simulink model "RBDmodel_unprotected"  (R2023a)
settings: Solver=ode15s  StartTime=0.0  StopTime=10  FixedStep=0.0001  RelTol=1e-3  AbsTol=1e-3  EnableMultiTasking=on
model workspace (MAT data in the model file):
  C_Gimbal = 0.1
  C_IAP = 0.01
  IAP_Pa = 0
  K_Gimbal = 0
  K_IAP = 0
  Left_EO = 0
  Left_IO = 0
  Left_MF = 0
  Left_RA = 0
  Moment_AR = 0
  Moment_FE = 7.5
  Moment_LB = 0
  Right_EO = 0
  Right_IO = 0
  Right_MF = 0
  Right_RA = 0
  a = 1
  b = 1
  muscle_color = [0 0 1]
  muscle_radius = 1
undefined symbols (not defined in the file): X, Y, Z
libraries: nesl_utility x346, sm_lib x329, simulink_extras x33, checkpacklib x3, simulink x1
(part 12 of 13)

== system RBDmodel_unprotected/subsystem/Segmental Moment-Rotation setup/L5-S1 AR setup ==
  Gain3 : Gain  Gain=-1
  Gain8 : Gain
  PS-Simulink Converter : nesl_utility/PS-Simulink Converter  PhysicalDomain=network_engine_domain  SubClassName=ps_output  LeftPortType=input  RightPortType=output  PseudoPeriodic=off  Frequencies=[]  VectorFormat=1-D array  Unit=rad  AffineConversion=off
  PS-Simulink Converter7 : nesl_utility/PS-Simulink Converter  PhysicalDomain=network_engine_domain  SubClassName=ps_output  LeftPortType=input  RightPortType=output  PseudoPeriodic=off  Frequencies=[]  VectorFormat=1-D array  Unit=N*m  AffineConversion=off
  Radians to Degrees : simulink_extras/Transformations/Radians to Degrees
  Moment : PMIOPort  Side=Left
  Rotation : PMIOPort  Port=2  Side=Left
  L5-S1 AR Simscape Rotation : Outport
  L5-S1 AR Simscape Moment : Outport  Port=2
  wires:
  Gain8/1 -> L5-S1 AR Simscape Moment/1  "L5-S1 AR Simscape Moment"
  PS-Simulink Converter7/1 -> Gain8/1
  Radians to Degrees/1 -> Gain3/1
  PS-Simulink Converter/1 -> Radians to Degrees/1
  Gain3/1 -> L5-S1 AR Simscape Rotation/1  "L5-S1 AR Simscape Rotation"
  connections:
  Rotation/RConn1 -- PS-Simulink Converter/LConn1
  Moment/RConn1 -- PS-Simulink Converter7/LConn1

== system RBDmodel_unprotected/subsystem/Segmental Moment-Rotation setup/L5-S1 FE setup ==
  Gain3 : Gain  Gain=-1
  Gain8 : Gain
  PS-Simulink Converter : nesl_utility/PS-Simulink Converter  PhysicalDomain=network_engine_domain  SubClassName=ps_output  LeftPortType=input  RightPortType=output  PseudoPeriodic=off  Frequencies=[]  VectorFormat=1-D array  Unit=rad  AffineConversion=off
  PS-Simulink Converter7 : nesl_utility/PS-Simulink Converter  PhysicalDomain=network_engine_domain  SubClassName=ps_output  LeftPortType=input  RightPortType=output  PseudoPeriodic=off  Frequencies=[]  VectorFormat=1-D array  Unit=N*m  AffineConversion=off
  Radians to Degrees : simulink_extras/Transformations/Radians to Degrees
  Moment : PMIOPort  Side=Left
  Rotation : PMIOPort  Port=2  Side=Left
  L5-S1 FE Simscape Rotation : Outport
  L5-S1 FE Simscape Moment : Outport  Port=2
  wires:
  Radians to Degrees/1 -> Gain3/1
  PS-Simulink Converter/1 -> Radians to Degrees/1
  PS-Simulink Converter7/1 -> Gain8/1
  Gain8/1 -> L5-S1 FE Simscape Moment/1  "L5-S1 FE Simscape Moment"
  Gain3/1 -> L5-S1 FE Simscape Rotation/1  "L5-S1 FE Simscape Rotation"
  connections:
  Rotation/RConn1 -- PS-Simulink Converter/LConn1
  Moment/RConn1 -- PS-Simulink Converter7/LConn1

== system RBDmodel_unprotected/subsystem/Segmental Moment-Rotation setup/L5-S1 LB setup ==
  Gain3 : Gain
  Gain8 : Gain  Gain=-1
  PS-Simulink Converter : nesl_utility/PS-Simulink Converter  PhysicalDomain=network_engine_domain  SubClassName=ps_output  LeftPortType=input  RightPortType=output  PseudoPeriodic=off  Frequencies=[]  VectorFormat=1-D array  Unit=rad  AffineConversion=off
  PS-Simulink Converter7 : nesl_utility/PS-Simulink Converter  PhysicalDomain=network_engine_domain  SubClassName=ps_output  LeftPortType=input  RightPortType=output  PseudoPeriodic=off  Frequencies=[]  VectorFormat=1-D array  Unit=N*m  AffineConversion=off
  Radians to Degrees : simulink_extras/Transformations/Radians to Degrees
  Moment : PMIOPort  Side=Left
  Rotation : PMIOPort  Port=2  Side=Left
  L5-S1 LB Simscape Rotation : Outport
  L5-S1 LB Simscape Moment : Outport  Port=2
  wires:
  Gain8/1 -> L5-S1 LB Simscape Moment/1  "L5-S1 LB Simscape Moment"
  PS-Simulink Converter/1 -> Radians to Degrees/1
  Radians to Degrees/1 -> Gain3/1
  Gain3/1 -> L5-S1 LB Simscape Rotation/1  "L5-S1 LB Simscape Rotation"
  PS-Simulink Converter7/1 -> Gain8/1
  connections:
  Moment/RConn1 -- PS-Simulink Converter7/LConn1
  Rotation/RConn1 -- PS-Simulink Converter/LConn1

== system RBDmodel_unprotected/subsystem/Segmental Moment-Rotation setup/Subsystem ==
  Gain3 : Gain  Gain=-1
  Gain8 : Gain
  PS-Simulink Converter : nesl_utility/PS-Simulink Converter  PhysicalDomain=network_engine_domain  SubClassName=ps_output  LeftPortType=input  RightPortType=output  PseudoPeriodic=off  Frequencies=[]  VectorFormat=1-D array  Unit=rad  AffineConversion=off
  PS-Simulink Converter7 : nesl_utility/PS-Simulink Converter  PhysicalDomain=network_engine_domain  SubClassName=ps_output  LeftPortType=input  RightPortType=output  PseudoPeriodic=off  Frequencies=[]  VectorFormat=1-D array  Unit=N*m  AffineConversion=off
  Radians to Degrees : simulink_extras/Transformations/Radians to Degrees
  Moment : PMIOPort  Side=Left
  Rotation : PMIOPort  Port=2  Side=Left
  L4-L5 FE Simscape Rotation : Outport
  L4-L5 FE Simscape Moment : Outport  Port=2
  wires:
  Radians to Degrees/1 -> Gain3/1
  PS-Simulink Converter/1 -> Radians to Degrees/1
  Gain8/1 -> L4-L5 FE Simscape Moment/1  "L4-L5 FE Simscape Moment"
  PS-Simulink Converter7/1 -> Gain8/1
  Gain3/1 -> L4-L5 FE Simscape Rotation/1  "L4-L5 FE Simscape Rotation"
  connections:
  Moment/RConn1 -- PS-Simulink Converter7/LConn1
  Rotation/RConn1 -- PS-Simulink Converter/LConn1

== system RBDmodel_unprotected/subsystem/Segmental Moment-Rotation setup/Subsystem1 ==
  Gain3 : Gain
  Gain8 : Gain  Gain=-1
  PS-Simulink Converter : nesl_utility/PS-Simulink Converter  PhysicalDomain=network_engine_domain  SubClassName=ps_output  LeftPortType=input  RightPortType=output  PseudoPeriodic=off  Frequencies=[]  VectorFormat=1-D array  Unit=rad  AffineConversion=off
  PS-Simulink Converter7 : nesl_utility/PS-Simulink Converter  PhysicalDomain=network_engine_domain  SubClassName=ps_output  LeftPortType=input  RightPortType=output  PseudoPeriodic=off  Frequencies=[]  VectorFormat=1-D array  Unit=N*m  AffineConversion=off
  Radians to Degrees : simulink_extras/Transformations/Radians to Degrees
  Moment : PMIOPort  Side=Left
  Rotation : PMIOPort  Port=2  Side=Left
  L4-L5 LB Simscape Rotation : Outport
  L4-L5 LB Simscape Moment : Outport  Port=2
  wires:
  PS-Simulink Converter/1 -> Radians to Degrees/1
  Gain3/1 -> L4-L5 LB Simscape Rotation/1  "L4-L5 LB Simscape Rotation"
  Radians to Degrees/1 -> Gain3/1
  PS-Simulink Converter7/1 -> Gain8/1
  Gain8/1 -> L4-L5 LB Simscape Moment/1  "L4-L5 LB Simscape Moment"
  connections:
  Rotation/RConn1 -- PS-Simulink Converter/LConn1
  Moment/RConn1 -- PS-Simulink Converter7/LConn1

== system RBDmodel_unprotected/subsystem/Segmental Moment-Rotation setup/Subsystem10 ==
  Gain3 : Gain
  Gain8 : Gain  Gain=-1
  PS-Simulink Converter : nesl_utility/PS-Simulink Converter  PhysicalDomain=network_engine_domain  SubClassName=ps_output  LeftPortType=input  RightPortType=output  PseudoPeriodic=off  Frequencies=[]  VectorFormat=1-D array  Unit=rad  AffineConversion=off
  PS-Simulink Converter7 : nesl_utility/PS-Simulink Converter  PhysicalDomain=network_engine_domain  SubClassName=ps_output  LeftPortType=input  RightPortType=output  PseudoPeriodic=off  Frequencies=[]  VectorFormat=1-D array  Unit=N*m  AffineConversion=off
  Radians to Degrees : simulink_extras/Transformations/Radians to Degrees
  Moment : PMIOPort  Side=Left
  Rotation : PMIOPort  Port=2  Side=Left
  L1-L2 LB Simscape Rotation : Outport
  L1-L2 LB Simscape Moment : Outport  Port=2
  wires:
  Radians to Degrees/1 -> Gain3/1
  PS-Simulink Converter/1 -> Radians to Degrees/1
  PS-Simulink Converter7/1 -> Gain8/1
  Gain3/1 -> L1-L2 LB Simscape Rotation/1  "L1-L2 LB Simscape Rotation"
  Gain8/1 -> L1-L2 LB Simscape Moment/1  "L1-L2 LB Simscape Moment"
  connections:
  Moment/RConn1 -- PS-Simulink Converter7/LConn1
  Rotation/RConn1 -- PS-Simulink Converter/LConn1

== system RBDmodel_unprotected/subsystem/Segmental Moment-Rotation setup/Subsystem11 ==
  Gain3 : Gain  Gain=-1
  Gain8 : Gain
  PS-Simulink Converter : nesl_utility/PS-Simulink Converter  PhysicalDomain=network_engine_domain  SubClassName=ps_output  LeftPortType=input  RightPortType=output  PseudoPeriodic=off  Frequencies=[]  VectorFormat=1-D array  Unit=rad  AffineConversion=off
  PS-Simulink Converter7 : nesl_utility/PS-Simulink Converter  PhysicalDomain=network_engine_domain  SubClassName=ps_output  LeftPortType=input  RightPortType=output  PseudoPeriodic=off  Frequencies=[]  VectorFormat=1-D array  Unit=N*m  AffineConversion=off
  Radians to Degrees : simulink_extras/Transformations/Radians to Degrees
  Moment : PMIOPort  Side=Left
  Rotation : PMIOPort  Port=2  Side=Left
  L1-L2 AR Simscape Rotation : Outport
  L1-L2 AR Simscape Moment : Outport  Port=2
  wires:
  Gain3/1 -> L1-L2 AR Simscape Rotation/1  "L1-L2 AR Simscape Rotation"
  Radians to Degrees/1 -> Gain3/1
  PS-Simulink Converter/1 -> Radians to Degrees/1
  PS-Simulink Converter7/1 -> Gain8/1
  Gain8/1 -> L1-L2 AR Simscape Moment/1  "L1-L2 AR Simscape Moment"
  connections:
  Moment/RConn1 -- PS-Simulink Converter7/LConn1
  Rotation/RConn1 -- PS-Simulink Converter/LConn1

== system RBDmodel_unprotected/subsystem/Segmental Moment-Rotation setup/Subsystem2 ==
  Gain3 : Gain  Gain=-1
  Gain8 : Gain
  PS-Simulink Converter : nesl_utility/PS-Simulink Converter  PhysicalDomain=network_engine_domain  SubClassName=ps_output  LeftPortType=input  RightPortType=output  PseudoPeriodic=off  Frequencies=[]  VectorFormat=1-D array  Unit=rad  AffineConversion=off
  PS-Simulink Converter7 : nesl_utility/PS-Simulink Converter  PhysicalDomain=network_engine_domain  SubClassName=ps_output  LeftPortType=input  RightPortType=output  PseudoPeriodic=off  Frequencies=[]  VectorFormat=1-D array  Unit=N*m  AffineConversion=off
  Radians to Degrees : simulink_extras/Transformations/Radians to Degrees
  Moment : PMIOPort  Side=Left
  Rotation : PMIOPort  Port=2  Side=Left
  L4-L5 AR Simscape Rotation : Outport
  L4-L5 AR Simscape Moment : Outport  Port=2
  wires:
  PS-Simulink Converter7/1 -> Gain8/1
  Radians to Degrees/1 -> Gain3/1
  Gain8/1 -> L4-L5 AR Simscape Moment/1  "L4-L5 AR Simscape Moment"
  PS-Simulink Converter/1 -> Radians to Degrees/1
  Gain3/1 -> L4-L5 AR Simscape Rotation/1  "L4-L5 AR Simscape Rotation"
  connections:
  Moment/RConn1 -- PS-Simulink Converter7/LConn1
  Rotation/RConn1 -- PS-Simulink Converter/LConn1

== system RBDmodel_unprotected/subsystem/Segmental Moment-Rotation setup/Subsystem3 ==
  Gain3 : Gain  Gain=-1
  Gain8 : Gain
  PS-Simulink Converter : nesl_utility/PS-Simulink Converter  PhysicalDomain=network_engine_domain  SubClassName=ps_output  LeftPortType=input  RightPortType=output  PseudoPeriodic=off  Frequencies=[]  VectorFormat=1-D array  Unit=rad  AffineConversion=off
  PS-Simulink Converter7 : nesl_utility/PS-Simulink Converter  PhysicalDomain=network_engine_domain  SubClassName=ps_output  LeftPortType=input  RightPortType=output  PseudoPeriodic=off  Frequencies=[]  VectorFormat=1-D array  Unit=N*m  AffineConversion=off
  Radians to Degrees : simulink_extras/Transformations/Radians to Degrees
  Moment : PMIOPort  Side=Left
  Rotation : PMIOPort  Port=2  Side=Left
  L3-L4 FE Simscape Rotation : Outport
  L3-L4 FE Simscape Moment : Outport  Port=2
  wires:
  Radians to Degrees/1 -> Gain3/1
  Gain3/1 -> L3-L4 FE Simscape Rotation/1  "L3-L4 FE Simscape Rotation"
  PS-Simulink Converter/1 -> Radians to Degrees/1
  PS-Simulink Converter7/1 -> Gain8/1
  Gain8/1 -> L3-L4 FE Simscape Moment/1  "L3-L4 FE Simscape Moment"
  connections:
  Moment/RConn1 -- PS-Simulink Converter7/LConn1
  Rotation/RConn1 -- PS-Simulink Converter/LConn1

== system RBDmodel_unprotected/subsystem/Segmental Moment-Rotation setup/Subsystem4 ==
  Gain3 : Gain
  Gain8 : Gain  Gain=-1
  PS-Simulink Converter : nesl_utility/PS-Simulink Converter  PhysicalDomain=network_engine_domain  SubClassName=ps_output  LeftPortType=input  RightPortType=output  PseudoPeriodic=off  Frequencies=[]  VectorFormat=1-D array  Unit=rad  AffineConversion=off
  PS-Simulink Converter7 : nesl_utility/PS-Simulink Converter  PhysicalDomain=network_engine_domain  SubClassName=ps_output  LeftPortType=input  RightPortType=output  PseudoPeriodic=off  Frequencies=[]  VectorFormat=1-D array  Unit=N*m  AffineConversion=off
  Radians to Degrees : simulink_extras/Transformations/Radians to Degrees
  Moment : PMIOPort  Side=Left
  Rotation : PMIOPort  Port=2  Side=Left
  L3-L4 LB Simscape Rotation : Outport
  L3-L4 LB Simscape Moment : Outport  Port=2
  wires:
  Gain8/1 -> L3-L4 LB Simscape Moment/1  "L3-L4 LB Simscape Moment"
  Radians to Degrees/1 -> Gain3/1
  PS-Simulink Converter/1 -> Radians to Degrees/1
  PS-Simulink Converter7/1 -> Gain8/1
  Gain3/1 -> L3-L4 LB Simscape Rotation/1  "L3-L4 LB Simscape Rotation"
  connections:
  Moment/RConn1 -- PS-Simulink Converter7/LConn1
  Rotation/RConn1 -- PS-Simulink Converter/LConn1

== system RBDmodel_unprotected/subsystem/Segmental Moment-Rotation setup/Subsystem5 ==
  Gain3 : Gain  Gain=-1
  Gain8 : Gain
  PS-Simulink Converter : nesl_utility/PS-Simulink Converter  PhysicalDomain=network_engine_domain  SubClassName=ps_output  LeftPortType=input  RightPortType=output  PseudoPeriodic=off  Frequencies=[]  VectorFormat=1-D array  Unit=rad  AffineConversion=off
  PS-Simulink Converter7 : nesl_utility/PS-Simulink Converter  PhysicalDomain=network_engine_domain  SubClassName=ps_output  LeftPortType=input  RightPortType=output  PseudoPeriodic=off  Frequencies=[]  VectorFormat=1-D array  Unit=N*m  AffineConversion=off
  Radians to Degrees : simulink_extras/Transformations/Radians to Degrees
  Moment : PMIOPort  Side=Left
  Rotation : PMIOPort  Port=2  Side=Left
  L3-L4 AR Simscape Rotation : Outport
  L3-L4 AR Simscape Moment : Outport  Port=2
  wires:
  PS-Simulink Converter/1 -> Radians to Degrees/1
  Gain8/1 -> L3-L4 AR Simscape Moment/1  "L3-L4 AR Simscape Moment"
  PS-Simulink Converter7/1 -> Gain8/1
  Radians to Degrees/1 -> Gain3/1
  Gain3/1 -> L3-L4 AR Simscape Rotation/1  "L3-L4 AR Simscape Rotation"
  connections:
  Moment/RConn1 -- PS-Simulink Converter7/LConn1
  Rotation/RConn1 -- PS-Simulink Converter/LConn1

== system RBDmodel_unprotected/subsystem/Segmental Moment-Rotation setup/Subsystem6 ==
  Gain3 : Gain  Gain=-1
  Gain8 : Gain
  PS-Simulink Converter : nesl_utility/PS-Simulink Converter  PhysicalDomain=network_engine_domain  SubClassName=ps_output  LeftPortType=input  RightPortType=output  PseudoPeriodic=off  Frequencies=[]  VectorFormat=1-D array  Unit=rad  AffineConversion=off
  PS-Simulink Converter7 : nesl_utility/PS-Simulink Converter  PhysicalDomain=network_engine_domain  SubClassName=ps_output  LeftPortType=input  RightPortType=output  PseudoPeriodic=off  Frequencies=[]  VectorFormat=1-D array  Unit=N*m  AffineConversion=off
  Radians to Degrees : simulink_extras/Transformations/Radians to Degrees
  Moment : PMIOPort  Side=Left
  Rotation : PMIOPort  Port=2  Side=Left
  L2-L3 FE Simscape Rotation : Outport
  L2-L3 FE Simscape Moment : Outport  Port=2
  wires:
  Gain3/1 -> L2-L3 FE Simscape Rotation/1  "L2-L3 FE Simscape Rotation"
  PS-Simulink Converter/1 -> Radians to Degrees/1
  PS-Simulink Converter7/1 -> Gain8/1
  Radians to Degrees/1 -> Gain3/1
  Gain8/1 -> L2-L3 FE Simscape Moment/1  "L2-L3 FE Simscape Moment"
  connections:
  Rotation/RConn1 -- PS-Simulink Converter/LConn1
  Moment/RConn1 -- PS-Simulink Converter7/LConn1

== system RBDmodel_unprotected/subsystem/Segmental Moment-Rotation setup/Subsystem7 ==
  Gain3 : Gain
  Gain8 : Gain  Gain=-1
  PS-Simulink Converter : nesl_utility/PS-Simulink Converter  PhysicalDomain=network_engine_domain  SubClassName=ps_output  LeftPortType=input  RightPortType=output  PseudoPeriodic=off  Frequencies=[]  VectorFormat=1-D array  Unit=rad  AffineConversion=off
  PS-Simulink Converter7 : nesl_utility/PS-Simulink Converter  PhysicalDomain=network_engine_domain  SubClassName=ps_output  LeftPortType=input  RightPortType=output  PseudoPeriodic=off  Frequencies=[]  VectorFormat=1-D array  Unit=N*m  AffineConversion=off
  Radians to Degrees : simulink_extras/Transformations/Radians to Degrees
  Moment : PMIOPort  Side=Left
  Rotation : PMIOPort  Port=2  Side=Left
  L2-L3 LB Simscape Rotation : Outport
  L2-L3 LB Simscape Moment : Outport  Port=2
  wires:
  PS-Simulink Converter7/1 -> Gain8/1
  PS-Simulink Converter/1 -> Radians to Degrees/1
  Radians to Degrees/1 -> Gain3/1
  Gain3/1 -> L2-L3 LB Simscape Rotation/1  "L2-L3 LB Simscape Rotation"
  Gain8/1 -> L2-L3 LB Simscape Moment/1  "L2-L3 LB Simscape Moment"
  connections:
  Rotation/RConn1 -- PS-Simulink Converter/LConn1
  Moment/RConn1 -- PS-Simulink Converter7/LConn1

== system RBDmodel_unprotected/subsystem/Segmental Moment-Rotation setup/Subsystem8 ==
  Gain3 : Gain  Gain=-1
  Gain8 : Gain
  PS-Simulink Converter : nesl_utility/PS-Simulink Converter  PhysicalDomain=network_engine_domain  SubClassName=ps_output  LeftPortType=input  RightPortType=output  PseudoPeriodic=off  Frequencies=[]  VectorFormat=1-D array  Unit=rad  AffineConversion=off
  PS-Simulink Converter7 : nesl_utility/PS-Simulink Converter  PhysicalDomain=network_engine_domain  SubClassName=ps_output  LeftPortType=input  RightPortType=output  PseudoPeriodic=off  Frequencies=[]  VectorFormat=1-D array  Unit=N*m  AffineConversion=off
  Radians to Degrees : simulink_extras/Transformations/Radians to Degrees
  Moment : PMIOPort  Side=Left
  Rotation : PMIOPort  Port=2  Side=Left
  L2-L3 AR Simscape Rotation : Outport
  L2-L3 AR Simscape Moment : Outport  Port=2
  wires:
  PS-Simulink Converter7/1 -> Gain8/1
  Radians to Degrees/1 -> Gain3/1
  PS-Simulink Converter/1 -> Radians to Degrees/1
  Gain3/1 -> L2-L3 AR Simscape Rotation/1  "L2-L3 AR Simscape Rotation"
  Gain8/1 -> L2-L3 AR Simscape Moment/1  "L2-L3 AR Simscape Moment"
  connections:
  Moment/RConn1 -- PS-Simulink Converter7/LConn1
  Rotation/RConn1 -- PS-Simulink Converter/LConn1

== system RBDmodel_unprotected/subsystem/Segmental Moment-Rotation setup/Subsystem9 ==
  Gain3 : Gain  Gain=-1
  Gain8 : Gain
  PS-Simulink Converter : nesl_utility/PS-Simulink Converter  PhysicalDomain=network_engine_domain  SubClassName=ps_output  LeftPortType=input  RightPortType=output  PseudoPeriodic=off  Frequencies=[]  VectorFormat=1-D array  Unit=rad  AffineConversion=off
  PS-Simulink Converter7 : nesl_utility/PS-Simulink Converter  PhysicalDomain=network_engine_domain  SubClassName=ps_output  LeftPortType=input  RightPortType=output  PseudoPeriodic=off  Frequencies=[]  VectorFormat=1-D array  Unit=N*m  AffineConversion=off
  Radians to Degrees : simulink_extras/Transformations/Radians to Degrees
  Moment : PMIOPort  Side=Left
  Rotation : PMIOPort  Port=2  Side=Left
  L1-L2 FE Simscape Rotation : Outport
  L1-L2 FE Simscape Moment : Outport  Port=2
  wires:
  PS-Simulink Converter/1 -> Radians to Degrees/1
  Gain3/1 -> L1-L2 FE Simscape Rotation/1  "L1-L2 FE Simscape Rotation"
  Gain8/1 -> L1-L2 FE Simscape Moment/1  "L1-L2 FE Simscape Moment"
  Radians to Degrees/1 -> Gain3/1
  PS-Simulink Converter7/1 -> Gain8/1
  connections:
  Rotation/RConn1 -- PS-Simulink Converter/LConn1
  Moment/RConn1 -- PS-Simulink Converter7/LConn1

== matlab function RBDmodel_unprotected/subsystem/L2/FE torque feedback L4/peacewise torque profile1 ==
  data: u input; torque output; a input; b input


function torque = T(u,a,b) % Guan et al logarithmic
    torque = 0;
    if (u >= 0)
     torque= a*(exp(u/8.23)-1)/0.10;

    elseif (u< 0)
     torque= b*(exp(u/-1.31)-1)/(-0.58)   ;
end

% function torque = T(u,a,b) % Rao et al segmental
%     torque = 0;
%     if (u >= 0)
%         torque= (a)*(-0.0042*u^2 + 1.9155*u);
%     elseif (u< 0)
%         torque= (b)*(-0.0042*u^2 + 1.9155*u);
% end

== matlab function RBDmodel_unprotected/subsystem/L2/LB torque feedback L4/peacewise torque profile4 ==
  data: u input; torque output; a input; b input
function torque = T(u,a,b)    % Guan et al (nonlinear logarithmic equation mentioned in their paper)
    torque = 0;
    if (u >= 0)
     torque= a*(exp(u/2.13)-1)/0.87;

    elseif (u< 0)
     torque= b*(exp(u/-2.22)-1)/(-0.66)   ;
end

== matlab function RBDmodel_unprotected/subsystem/L1/AR torque feedback L4/peacewise torque profile5 ==
  data: u input; torque output; a input; b input
function torque = T(u,a,b)    % Panjabi data fitted into logarithmic equation. Refer validation.xlsx
    torque = 0;
    if (u >= 0)
     torque= a*(exp(u/0.83)-1)/0.35;

    elseif (u < 0)
     torque= b*(exp(u/-0.38)-1)/(-3.18)   ;
end

== matlab function RBDmodel_unprotected/subsystem/L1/FE torque feedback L4/peacewise torque profile1 ==
  data: u input; torque output; a input; b input
% function torque = T(u,udot)  % Guan et al logarithmic plus  (RECALCULATED - refer excel)
%     torque = 0;
%     if (u >= 0)
%      torque= (exp(u/8.067)-1)/0.1031   +    0.1*udot;
% 
%     elseif (u < 0)
%      torque= (exp(u/-1.2951)-1)/(-0.5753) +  0.1*udot  ;
% end



function torque = T(u,a,b)  % Guan et al logarithmic  (RECALCULATED - refer excel)
    torque = 0;
    if (u >= 0)
     torque= a*(exp(u/8.067)-1)/0.1031;

    elseif (u < 0)
     torque= b*(exp(u/-1.2951)-1)/(-0.5753)   ;
end


% function torque = T(u,a,b)  % Rao et al segmental
%     torque = 0;
%     if (u >= 0)
%         torque = (a)*(0.0343*u^2 + 1.9989*u);
%     elseif (u < 0)
%         torque = (b)*(0.0343*u^2 + 1.9989*u);
% end

== matlab function RBDmodel_unprotected/subsystem/L1/LB torque feedback L4/peacewise torque profile4 ==
  data: u input; torque output; a input; b input
function torque = T(u,a,b)    % Guan et al (RECALCULATED - refer excel)
    torque = 0;
    if (u >= 0)
     torque= a*(exp(u/2.0545)-1)/0.9457;

    elseif (u< 0)
     torque= b*(exp(u/-2.3716)-1)/(-0.5744)   ;
end

== matlab function RBDmodel_unprotected/Muscle force inputs/Sum of Square of Forces ==
  data: F1 input; SumofSquareofForces output; F2 input; F3 input; F4 input; F5 input; F6 input; F7 input; F8 input; IAP input
function SumofSquareofForces = fcn(F1,F2,F3,F4,F5,F6,F7,F8,IAP)

SumofSquareofForces = F1^2 + F2^2 + F3^2 + F4^2 + F5^2 + F6^2 +F7^2 + F8^2 + IAP^2;

== matlab function RBDmodel_unprotected/subsystem/L4/FE torque feedback L4/peacewise torque profile1 ==
  data: u input; torque output; a input; b input


function torque = T(u,a,b) % Guan et al logarithmic
    torque = 0;
    if (u >= 0)
     torque= a*(exp(u/3.07)-1)/0.81;

    elseif (u< 0)
     torque= b*(exp(u/-8.14)-1)/(-0.05)   ;
end

% function torque = T(u,a,b) % Rao et al segmental
%     torque = 0;
%     if (u >= 0)
%         torque= (a)*(0.0493*u^2 + 2.2629*u);
%     elseif (u< 0)
%         torque= (b)*(0.0493*u^2 + 2.2629*u);
% end

== matlab function RBDmodel_unprotected/subsystem/Spinal Kinematics Setup/MATLAB Function ==
  data: y input; angle output; z input
function angle = fcn(y,z)

angle = 90 - (57.2958*atan(z/y));

end

== matlab function RBDmodel_unprotected/subsystem/Muscle Forces setup/Muscle2/MATLAB Function2 ==
  data: x1 input; length output; y1 input; z1 input; x2 input; y2 input; z2 input; Rx output; Ry output; Rz output
function [length, Rx, Ry, Rz] = computeCylinderParameters(x1, y1, z1, x2, y2, z2)
    % Compute the vector between the two frames
    vector = [x2 - x1, y2 - y1, z2 - z1];
    
    % Compute the length of the cylinder
    length = norm(vector);
    
    % Normalize the vector for direction
    unit_vector = vector / length;
    
    % Assume fixed axis (Z-axis)
    fixed_axis = [0, 0, 1];
    
    % Compute the axis of rotation (cross product)
    axis_of_rotation = cross(unit_vector, fixed_axis);
    
    % Avoid division by zero in case vectors are parallel
    if norm(axis_of_rotation) == 0
        % Handle case when the vectors are parallel
        if dot(unit_vector, fixed_axis) > 0
            % Vectors are aligned, no rotation needed
            Rx = 0;
            Ry = 0;
            Rz = 0;
        else
            % Vectors are in opposite directions, 180 degree rotation
            Rx = pi;
            Ry = 0;
            Rz = 0;
        end
        return;
    end
    
    % Normalize the axis of rotation
    axis_of_rotation = axis_of_rotation / norm(axis_of_rotation);
    
    % Compute the angle between vectors (dot product)
    cos_theta = dot(unit_vector, fixed_axis);
    
    % Clamp cos_theta to the range [-1, 1] to avoid domain errors in acos
    cos_theta = max(min(cos_theta, 1), -1);
    angle = acos(cos_theta);  % The angle between the vectors
    
    % Rodrigues' rotation formula to compute the rotation matrix
    K = [0, -axis_of_rotation(3), axis_of_rotation(2); 
         axis_of_rotation(3), 0, -axis_of_rotation(1); 
         -axis_of_rotation(2), axis_of_rotation(1), 0]; 
    R = eye(3) + sin(angle)*K + (1 - cos(angle))*(K^2);
    
    % Now, decompose the rotation matrix to extract the Euler angles
    Rx = -atan2(R(3,2), R(3,3)); % Rotation about X-axis
    %Ry = atan2(-R(3,1), sqrt(R(3,2)^2 + R(3,3)^2)); % Rotation about Y-axis
    denominator = max(sqrt(R(3,2)^2 + R(3,3)^2), eps); % Avoid division by zero
    Ry = -atan2(-R(3,1), denominator);

    
    
    Rz = 0; % No additional rotation needed around the Z-axis
end

== matlab function RBDmodel_unprotected/subsystem/Muscle Forces setup/Muscle3/MATLAB Function2 ==
  data: x1 input; length output; y1 input; z1 input; x2 input; y2 input; z2 input; Rx output; Ry output; Rz output
function [length, Rx, Ry, Rz] = computeCylinderParameters(x1, y1, z1, x2, y2, z2)
    % Compute the vector between the two frames
    vector = [x2 - x1, y2 - y1, z2 - z1];
    
    % Compute the length of the cylinder
    length = norm(vector);
    
    % Normalize the vector for direction
    unit_vector = vector / length;
    
    % Assume fixed axis (Z-axis)
    fixed_axis = [0, 0, 1];
    
    % Compute the axis of rotation (cross product)
    axis_of_rotation = cross(unit_vector, fixed_axis);
    
    % Avoid division by zero in case vectors are parallel
    if norm(axis_of_rotation) == 0
        % Handle case when the vectors are parallel
        if dot(unit_vector, fixed_axis) > 0
            % Vectors are aligned, no rotation needed
            Rx = 0;
            Ry = 0;
            Rz = 0;
        else
            % Vectors are in opposite directions, 180 degree rotation
            Rx = pi;
            Ry = 0;
            Rz = 0;
        end
        return;
    end
    
    % Normalize the axis of rotation
    axis_of_rotation = axis_of_rotation / norm(axis_of_rotation);
    
    % Compute the angle between vectors (dot product)
    cos_theta = dot(unit_vector, fixed_axis);
    
    % Clamp cos_theta to the range [-1, 1] to avoid domain errors in acos
    cos_theta = max(min(cos_theta, 1), -1);
    angle = acos(cos_theta);  % The angle between the vectors
    
    % Rodrigues' rotation formula to compute the rotation matrix
    K = [0, -axis_of_rotation(3), axis_of_rotation(2); 
         axis_of_rotation(3), 0, -axis_of_rotation(1); 
         -axis_of_rotation(2), axis_of_rotation(1), 0]; 
    R = eye(3) + sin(angle)*K + (1 - cos(angle))*(K^2);
    
    % Now, decompose the rotation matrix to extract the Euler angles
    Rx = -atan2(R(3,2), R(3,3)); % Rotation about X-axis
    %Ry = atan2(-R(3,1), sqrt(R(3,2)^2 + R(3,3)^2)); % Rotation about Y-axis
    denominator = max(sqrt(R(3,2)^2 + R(3,3)^2), eps); % Avoid division by zero
    Ry = -atan2(-R(3,1), denominator);

    
    
    Rz = 0; % No additional rotation needed around the Z-axis
end

== matlab function RBDmodel_unprotected/subsystem/Muscle Forces setup/Muscle1/MATLAB Function2 ==
  data: x1 input; length output; y1 input; z1 input; x2 input; y2 input; z2 input; Rx output; Ry output; Rz output
function [length, Rx, Ry, Rz] = computeCylinderParameters(x1, y1, z1, x2, y2, z2)
    % Compute the vector between the two frames
    vector = [x2 - x1, y2 - y1, z2 - z1];
    
    % Compute the length of the cylinder
    length = norm(vector);
    
    % Normalize the vector for direction
    unit_vector = vector / length;
    
    % Assume fixed axis (Z-axis)
    fixed_axis = [0, 0, 1];
    
    % Compute the axis of rotation (cross product)
    axis_of_rotation = cross(unit_vector, fixed_axis);
    
    % Avoid division by zero in case vectors are parallel
    if norm(axis_of_rotation) == 0
        % Handle case when the vectors are parallel
        if dot(unit_vector, fixed_axis) > 0
            % Vectors are aligned, no rotation needed
            Rx = 0;
            Ry = 0;
            Rz = 0;
        else
            % Vectors are in opposite directions, 180 degree rotation
            Rx = pi;
            Ry = 0;
            Rz = 0;
        end
        return;
    end
    
    % Normalize the axis of rotation
    axis_of_rotation = axis_of_rotation / norm(axis_of_rotation);
    
    % Compute the angle between vectors (dot product)
    cos_theta = dot(unit_vector, fixed_axis);
    
    % Clamp cos_theta to the range [-1, 1] to avoid domain errors in acos
    cos_theta = max(min(cos_theta, 1), -1);
    angle = acos(cos_theta);  % The angle between the vectors
    
    % Rodrigues' rotation formula to compute the rotation matrix
    K = [0, -axis_of_rotation(3), axis_of_rotation(2); 
         axis_of_rotation(3), 0, -axis_of_rotation(1); 
         -axis_of_rotation(2), axis_of_rotation(1), 0]; 
    R = eye(3) + sin(angle)*K + (1 - cos(angle))*(K^2);
    
    % Now, decompose the rotation matrix to extract the Euler angles
    Rx = -atan2(R(3,2), R(3,3)); % Rotation about X-axis
    %Ry = atan2(-R(3,1), sqrt(R(3,2)^2 + R(3,3)^2)); % Rotation about Y-axis
    denominator = max(sqrt(R(3,2)^2 + R(3,3)^2), eps); % Avoid division by zero
    Ry = -atan2(-R(3,1), denominator);

    
    
    Rz = 0; % No additional rotation needed around the Z-axis
end

== matlab function RBDmodel_unprotected/subsystem/Muscle Forces setup/Muscle4/MATLAB Function2 ==
  data: x1 input; length output; y1 input; z1 input; x2 input; y2 input; z2 input; Rx output; Ry output; Rz output
function [length, Rx, Ry, Rz] = computeCylinderParameters(x1, y1, z1, x2, y2, z2)
    % Compute the vector between the two frames
    vector = [x2 - x1, y2 - y1, z2 - z1];
    
    % Compute the length of the cylinder
    length = norm(vector);
    
    % Normalize the vector for direction
    unit_vector = vector / length;
    
    % Assume fixed axis (Z-axis)
    fixed_axis = [0, 0, 1];
    
    % Compute the axis of rotation (cross product)
    axis_of_rotation = cross(unit_vector, fixed_axis);
    
    % Avoid division by zero in case vectors are parallel
    if norm(axis_of_rotation) == 0
        % Handle case when the vectors are parallel
        if dot(unit_vector, fixed_axis) > 0
            % Vectors are aligned, no rotation needed
            Rx = 0;
            Ry = 0;
            Rz = 0;
        else
            % Vectors are in opposite directions, 180 degree rotation
            Rx = pi;
            Ry = 0;
            Rz = 0;
        end
        return;
    end
    
    % Normalize the axis of rotation
    axis_of_rotation = axis_of_rotation / norm(axis_of_rotation);
    
    % Compute the angle between vectors (dot product)
    cos_theta = dot(unit_vector, fixed_axis);
    
    % Clamp cos_theta to the range [-1, 1] to avoid domain errors in acos
    cos_theta = max(min(cos_theta, 1), -1);
    angle = acos(cos_theta);  % The angle between the vectors
    
    % Rodrigues' rotation formula to compute the rotation matrix
    K = [0, -axis_of_rotation(3), axis_of_rotation(2); 
         axis_of_rotation(3), 0, -axis_of_rotation(1); 
         -axis_of_rotation(2), axis_of_rotation(1), 0]; 
    R = eye(3) + sin(angle)*K + (1 - cos(angle))*(K^2);
    
    % Now, decompose the rotation matrix to extract the Euler angles
    Rx = -atan2(R(3,2), R(3,3)); % Rotation about X-axis
    %Ry = atan2(-R(3,1), sqrt(R(3,2)^2 + R(3,3)^2)); % Rotation about Y-axis
    denominator = max(sqrt(R(3,2)^2 + R(3,3)^2), eps); % Avoid division by zero
    Ry = -atan2(-R(3,1), denominator);

    
    
    Rz = 0; % No additional rotation needed around the Z-axis
end

== matlab function RBDmodel_unprotected/subsystem/Muscle Forces setup/Muscle5/MATLAB Function2 ==
  data: x1 input; length output; y1 input; z1 input; x2 input; y2 input; z2 input; Rx output; Ry output; Rz output
function [length, Rx, Ry, Rz] = computeCylinderParameters(x1, y1, z1, x2, y2, z2)
    % Compute the vector between the two frames
    vector = [x2 - x1, y2 - y1, z2 - z1];
    
    % Compute the length of the cylinder
    length = norm(vector);
    
    % Normalize the vector for direction
    unit_vector = vector / length;
    
    % Assume fixed axis (Z-axis)
    fixed_axis = [0, 0, 1];
    
    % Compute the axis of rotation (cross product)
    axis_of_rotation = cross(unit_vector, fixed_axis);
    
    % Avoid division by zero in case vectors are parallel
    if norm(axis_of_rotation) == 0
        % Handle case when the vectors are parallel
        if dot(unit_vector, fixed_axis) > 0
            % Vectors are aligned, no rotation needed
            Rx = 0;
            Ry = 0;
            Rz = 0;
        else
            % Vectors are in opposite directions, 180 degree rotation
            Rx = pi;
            Ry = 0;
            Rz = 0;
        end
        return;
    end
    
    % Normalize the axis of rotation
    axis_of_rotation = axis_of_rotation / norm(axis_of_rotation);
    
    % Compute the angle between vectors (dot product)
    cos_theta = dot(unit_vector, fixed_axis);
    
    % Clamp cos_theta to the range [-1, 1] to avoid domain errors in acos
    cos_theta = max(min(cos_theta, 1), -1);
    angle = acos(cos_theta);  % The angle between the vectors
    
    % Rodrigues' rotation formula to compute the rotation matrix
    K = [0, -axis_of_rotation(3), axis_of_rotation(2); 
         axis_of_rotation(3), 0, -axis_of_rotation(1); 
         -axis_of_rotation(2), axis_of_rotation(1), 0]; 
    R = eye(3) + sin(angle)*K + (1 - cos(angle))*(K^2);
    
    % Now, decompose the rotation matrix to extract the Euler angles
    Rx = -atan2(R(3,2), R(3,3)); % Rotation about X-axis
    %Ry = atan2(-R(3,1), sqrt(R(3,2)^2 + R(3,3)^2)); % Rotation about Y-axis
    denominator = max(sqrt(R(3,2)^2 + R(3,3)^2), eps); % Avoid division by zero
    Ry = -atan2(-R(3,1), denominator);

    
    
    Rz = 0; % No additional rotation needed around the Z-axis
end

== matlab function RBDmodel_unprotected/subsystem/Muscle Forces setup/Muscle6/MATLAB Function2 ==
  data: x1 input; length output; y1 input; z1 input; x2 input; y2 input; z2 input; Rx output; Ry output; Rz output
function [length, Rx, Ry, Rz] = computeCylinderParameters(x1, y1, z1, x2, y2, z2)
    % Compute the vector between the two frames
    vector = [x2 - x1, y2 - y1, z2 - z1];
    
    % Compute the length of the cylinder
    length = norm(vector);
    
    % Normalize the vector for direction
    unit_vector = vector / length;
    
    % Assume fixed axis (Z-axis)
    fixed_axis = [0, 0, 1];
    
    % Compute the axis of rotation (cross product)
    axis_of_rotation = cross(unit_vector, fixed_axis);
    
    % Avoid division by zero in case vectors are parallel
    if norm(axis_of_rotation) == 0
        % Handle case when the vectors are parallel
        if dot(unit_vector, fixed_axis) > 0
            % Vectors are aligned, no rotation needed
            Rx = 0;
            Ry = 0;
            Rz = 0;
        else
            % Vectors are in opposite directions, 180 degree rotation
            Rx = pi;
            Ry = 0;
            Rz = 0;
        end
        return;
    end
    
    % Normalize the axis of rotation
    axis_of_rotation = axis_of_rotation / norm(axis_of_rotation);
    
    % Compute the angle between vectors (dot product)
    cos_theta = dot(unit_vector, fixed_axis);
    
    % Clamp cos_theta to the range [-1, 1] to avoid domain errors in acos
    cos_theta = max(min(cos_theta, 1), -1);
    angle = acos(cos_theta);  % The angle between the vectors
    
    % Rodrigues' rotation formula to compute the rotation matrix
    K = [0, -axis_of_rotation(3), axis_of_rotation(2); 
         axis_of_rotation(3), 0, -axis_of_rotation(1); 
         -axis_of_rotation(2), axis_of_rotation(1), 0]; 
    R = eye(3) + sin(angle)*K + (1 - cos(angle))*(K^2);
    
    % Now, decompose the rotation matrix to extract the Euler angles
    Rx = -atan2(R(3,2), R(3,3)); % Rotation about X-axis
    %Ry = atan2(-R(3,1), sqrt(R(3,2)^2 + R(3,3)^2)); % Rotation about Y-axis
    denominator = max(sqrt(R(3,2)^2 + R(3,3)^2), eps); % Avoid division by zero
    Ry = -atan2(-R(3,1), denominator);

    
    
    Rz = 0; % No additional rotation needed around the Z-axis
end

== matlab function RBDmodel_unprotected/subsystem/L5/FE torque feedback L5/peacewise torque profile (+- 15 deg) ==
  data: u input; torque output; a input; b input


function torque = T(u,a,b)    % Guan et al (nonlinear logarithmic equation mentioned in their paper)
    torque = 0;
    if (u >= 0)
     torque= a*(exp(u/5.58)-1)/0.59;

    elseif (u< 0)
     torque= b*(exp(u/-4.48)-1)/(-0.33)   ;
end

% function torque = T(u,a,b)    % Rao et al segmental data
%     torque = 0;
%     if (u >= 0)
%         torque= (a)*(0.0348*u^3 + 0.089*u^2 + 1.1837*u);
%     elseif (u< 0)
%         torque= (b)*(0.0348*u^3 + 0.089*u^2 + 1.1837*u);
% end

== matlab function RBDmodel_unprotected/subsystem/Muscle Forces setup/Muscle7/MATLAB Function2 ==
  data: x1 input; length output; y1 input; z1 input; x2 input; y2 input; z2 input; Rx output; Ry output; Rz output
function [length, Rx, Ry, Rz] = computeCylinderParameters(x1, y1, z1, x2, y2, z2)
    % Compute the vector between the two frames
    vector = [x2 - x1, y2 - y1, z2 - z1];
    
    % Compute the length of the cylinder
    length = norm(vector);
    
    % Normalize the vector for direction
    unit_vector = vector / length;
    
    % Assume fixed axis (Z-axis)
    fixed_axis = [0, 0, 1];
    
    % Compute the axis of rotation (cross product)
    axis_of_rotation = cross(unit_vector, fixed_axis);
    
    % Avoid division by zero in case vectors are parallel
    if norm(axis_of_rotation) == 0
        % Handle case when the vectors are parallel
        if dot(unit_vector, fixed_axis) > 0
            % Vectors are aligned, no rotation needed
            Rx = 0;
            Ry = 0;
            Rz = 0;
        else
            % Vectors are in opposite directions, 180 degree rotation
            Rx = pi;
            Ry = 0;
            Rz = 0;
        end
        return;
    end
    
    % Normalize the axis of rotation
    axis_of_rotation = axis_of_rotation / norm(axis_of_rotation);
    
    % Compute the angle between vectors (dot product)
    cos_theta = dot(unit_vector, fixed_axis);
    
    % Clamp cos_theta to the range [-1, 1] to avoid domain errors in acos
    cos_theta = max(min(cos_theta, 1), -1);
    angle = acos(cos_theta);  % The angle between the vectors
    
    % Rodrigues' rotation formula to compute the rotation matrix
    K = [0, -axis_of_rotation(3), axis_of_rotation(2); 
         axis_of_rotation(3), 0, -axis_of_rotation(1); 
         -axis_of_rotation(2), axis_of_rotation(1), 0]; 
    R = eye(3) + sin(angle)*K + (1 - cos(angle))*(K^2);
    
    % Now, decompose the rotation matrix to extract the Euler angles
    Rx = -atan2(R(3,2), R(3,3)); % Rotation about X-axis
    %Ry = atan2(-R(3,1), sqrt(R(3,2)^2 + R(3,3)^2)); % Rotation about Y-axis
    denominator = max(sqrt(R(3,2)^2 + R(3,3)^2), eps); % Avoid division by zero
    Ry = -atan2(-R(3,1), denominator);

    
    
    Rz = 0; % No additional rotation needed around the Z-axis
end

== matlab function RBDmodel_unprotected/subsystem/Muscle Forces setup/Muscle8/MATLAB Function2 ==
  data: x1 input; length output; y1 input; z1 input; x2 input; y2 input; z2 input; Rx output; Ry output; Rz output
function [length, Rx, Ry, Rz] = computeCylinderParameters(x1, y1, z1, x2, y2, z2)
    % Compute the vector between the two frames
    vector = [x2 - x1, y2 - y1, z2 - z1];
    
    % Compute the length of the cylinder
    length = norm(vector);
    
    % Normalize the vector for direction
    unit_vector = vector / length;
    
    % Assume fixed axis (Z-axis)
    fixed_axis = [0, 0, 1];
    
    % Compute the axis of rotation (cross product)
    axis_of_rotation = cross(unit_vector, fixed_axis);
    
    % Avoid division by zero in case vectors are parallel
    if norm(axis_of_rotation) == 0
        % Handle case when the vectors are parallel
        if dot(unit_vector, fixed_axis) > 0
            % Vectors are aligned, no rotation needed
            Rx = 0;
            Ry = 0;
            Rz = 0;
        else
            % Vectors are in opposite directions, 180 degree rotation
            Rx = pi;
            Ry = 0;
            Rz = 0;
        end
        return;
    end
    
    % Normalize the axis of rotation
    axis_of_rotation = axis_of_rotation / norm(axis_of_rotation);
    
    % Compute the angle between vectors (dot product)
    cos_theta = dot(unit_vector, fixed_axis);
    
    % Clamp cos_theta to the range [-1, 1] to avoid domain errors in acos
    cos_theta = max(min(cos_theta, 1), -1);
    angle = acos(cos_theta);  % The angle between the vectors
    
    % Rodrigues' rotation formula to compute the rotation matrix
    K = [0, -axis_of_rotation(3), axis_of_rotation(2); 
         axis_of_rotation(3), 0, -axis_of_rotation(1); 
         -axis_of_rotation(2), axis_of_rotation(1), 0]; 
    R = eye(3) + sin(angle)*K + (1 - cos(angle))*(K^2);
    
    % Now, decompose the rotation matrix to extract the Euler angles
    Rx = -atan2(R(3,2), R(3,3)); % Rotation about X-axis
    %Ry = atan2(-R(3,1), sqrt(R(3,2)^2 + R(3,3)^2)); % Rotation about Y-axis
    denominator = max(sqrt(R(3,2)^2 + R(3,3)^2), eps); % Avoid division by zero
    Ry = -atan2(-R(3,1), denominator);

    
    
    Rz = 0; % No additional rotation needed around the Z-axis
end

== matlab function RBDmodel_unprotected/subsystem/Muscle Forces setup/WrapedMuscle/MATLAB Function2 ==
  data: x1 input; length output; y1 input; z1 input; x2 input; y2 input; z2 input; Rx output; Ry output; Rz output
function [length, Rx, Ry, Rz] = computeCylinderParameters(x1, y1, z1, x2, y2, z2)
    % Compute the vector between the two frames
    vector = [x2 - x1, y2 - y1, z2 - z1];
    
    % Compute the length of the cylinder
    length = norm(vector);
    
    % Normalize the vector for direction
    unit_vector = vector / length;
    
    % Assume fixed axis (Z-axis)
    fixed_axis = [0, 0, 1];
    
    % Compute the axis of rotation (cross product)
    axis_of_rotation = cross(unit_vector, fixed_axis);
    
    % Avoid division by zero in case vectors are parallel
    if norm(axis_of_rotation) == 0
        % Handle case when the vectors are parallel
        if dot(unit_vector, fixed_axis) > 0
            % Vectors are aligned, no rotation needed
            Rx = 0;
            Ry = 0;
            Rz = 0;
        else
            % Vectors are in opposite directions, 180 degree rotation
            Rx = pi;
            Ry = 0;
            Rz = 0;
        end
        return;
    end
    
    % Normalize the axis of rotation
    axis_of_rotation = axis_of_rotation / norm(axis_of_rotation);
    
    % Compute the angle between vectors (dot product)
    cos_theta = dot(unit_vector, fixed_axis);
    
    % Clamp cos_theta to the range [-1, 1] to avoid domain errors in acos
    cos_theta = max(min(cos_theta, 1), -1);
    angle = acos(cos_theta);  % The angle between the vectors
    
    % Rodrigues' rotation formula to compute the rotation matrix
    K = [0, -axis_of_rotation(3), axis_of_rotation(2); 
         axis_of_rotation(3), 0, -axis_of_rotation(1); 
         -axis_of_rotation(2), axis_of_rotation(1), 0]; 
    R = eye(3) + sin(angle)*K + (1 - cos(angle))*(K^2);
    
    % Now, decompose the rotation matrix to extract the Euler angles
    Rx = -atan2(R(3,2), R(3,3)); % Rotation about X-axis
    %Ry = atan2(-R(3,1), sqrt(R(3,2)^2 + R(3,3)^2)); % Rotation about Y-axis
    denominator = max(sqrt(R(3,2)^2 + R(3,3)^2), eps); % Avoid division by zero
    Ry = -atan2(-R(3,1), denominator);

    
    
    Rz = 0; % No additional rotation needed around the Z-axis
end

== matlab function RBDmodel_unprotected/subsystem/Muscle Forces setup/WrapedMuscle/MATLAB Function1 ==
  data: x1 input; length output; y1 input; z1 input; x2 input; y2 input; z2 input; Rx output; Ry output; Rz output
function [length, Rx, Ry, Rz] = computeCylinderParameters(x1, y1, z1, x2, y2, z2)
    % Compute the vector between the two frames
    vector = [x2 - x1, y2 - y1, z2 - z1];
    
    % Compute the length of the cylinder
    length = norm(vector);
    
    % Normalize the vector for direction
    unit_vector = vector / length;
    
    % Assume fixed axis (Z-axis)
    fixed_axis = [0, 0, 1];
    
    % Compute the axis of rotation (cross product)
    axis_of_rotation = cross(unit_vector, fixed_axis);
    
    % Avoid division by zero in case vectors are parallel
    if norm(axis_of_rotation) == 0
        % Handle case when the vectors are parallel
        if dot(unit_vector, fixed_axis) > 0
            % Vectors are aligned, no rotation needed
            Rx = 0;
            Ry = 0;
            Rz = 0;
        else
            % Vectors are in opposite directions, 180 degree rotation
            Rx = pi;
            Ry = 0;
            Rz = 0;
        end
        return;
    end
    
    % Normalize the axis of rotation
    axis_of_rotation = axis_of_rotation / norm(axis_of_rotation);
    
    % Compute the angle between vectors (dot product)
    cos_theta = dot(unit_vector, fixed_axis);
    
    % Clamp cos_theta to the range [-1, 1] to avoid domain errors in acos
    cos_theta = max(min(cos_theta, 1), -1);
    angle = acos(cos_theta);  % The angle between the vectors
    
    % Rodrigues' rotation formula to compute the rotation matrix
    K = [0, -axis_of_rotation(3), axis_of_rotation(2); 
         axis_of_rotation(3), 0, -axis_of_rotation(1); 
         -axis_of_rotation(2), axis_of_rotation(1), 0]; 
    R = eye(3) + sin(angle)*K + (1 - cos(angle))*(K^2);
    
    % Now, decompose the rotation matrix to extract the Euler angles
    Rx = -atan2(R(3,2), R(3,3)); % Rotation about X-axis
    %Ry = atan2(-R(3,1), sqrt(R(3,2)^2 + R(3,3)^2)); % Rotation about Y-axis
    denominator = max(sqrt(R(3,2)^2 + R(3,3)^2), eps); % Avoid division by zero
    Ry = -atan2(-R(3,1), denominator);

    
    
    Rz = 0; % No additional rotation needed around the Z-axis
end

== matlab function RBDmodel_unprotected/subsystem/L5/LB torque feedback L5/peacewise torque profile2 ==
  data: u input; torque output; a input; b input
function torque = T(u,a,b)    % Guan et al (nonlinear logarithmic equation mentioned in their paper)
    torque = 0;
    if (u >= 0)
     torque= a*(exp(u/3.26)-1)/0.49;

    elseif (u < 0)
     torque= b*(exp(u/-4.22)-1)/(-0.29)   ;
end

== matlab function RBDmodel_unprotected/subsystem/L5/AR torque feedback L5/peacewise torque profile3 ==
  data: u input; torque output; a input; b input
function torque = T(u,a,b)    % Panjabi data fitted into logarithmic equation. Refer validation.xlsx
    torque = 0;
    if (u >= 0)
     torque= a*(exp(u/1.25)-1)/0.10;

    elseif (u < 0)
     torque= b*(exp(u/-1.05)-1)/(-0.10)   ;
end

== matlab function RBDmodel_unprotected/subsystem/L4/LB torque feedback L4/peacewise torque profile4 ==
  data: u input; torque output; a input; b input
function torque = T(u,a,b)    % Guan et al (nonlinear logarithmic equation mentioned in their paper)
    torque = 0;
    if (u >= 0)
     torque= a*(exp(u/1.77)-1)/1.28;

    elseif (u< 0)
     torque= b*(exp(u/-1.44)-1)/(-1.23)   ;
end

== matlab function RBDmodel_unprotected/subsystem/L4/AR torque feedback L4/peacewise torque profile5 ==
  data: u input; torque output; a input; b input
function torque = T(u,a,b)    % Panjabi data fitted into logarithmic equation. Refer validation.xlsx
    torque = 0;
    if (u >= 0)
     torque= a*(exp(u/0.73)-1)/0.20;

    elseif (u < 0)
     torque= b*(exp(u/-1.01)-1)/(-0.31)   ;
end

== matlab function RBDmodel_unprotected/subsystem/L3/AR torque feedback L4/peacewise torque profile5 ==
  data: u input; torque output; a input; b input
function torque = T(u,a,b)    % Panjabi data fitted into logarithmic equation. Refer validation.xlsx
    torque = 0;
    if (u >= 0)
     torque= a*(exp(u/2.69)-1)/0.10;

    elseif (u < 0)
     torque= b*(exp(u/-0.90)-1)/(-0.89)   ;
end

== matlab function RBDmodel_unprotected/subsystem/L3/FE torque feedback L4/peacewise torque profile1 ==
  data: u input; torque output; a input; b input

function torque = T(u,a,b)  % Guan et al logarithmic
    torque = 0;
    if (u >= 0)
     torque= a*(exp(u/11.09)-1)/0.09;

    elseif (u< 0)
     torque= b*(exp(u/-24.35)-1)/(-0.02)   ;
end

% function torque = T(u,a,b)  % Rao et al segmental
%     torque = 0;
%     if (u >= 0)
%         torque = (a)*(0.0342*u^3 + 0.0596*u^2 + 1.5861*u);
%     elseif (u< 0)
%         torque = (b)*(0.0342*u^3 + 0.0596*u^2 + 1.5861*u);
% end

== matlab function RBDmodel_unprotected/subsystem/L3/LB torque feedback L4/peacewise torque profile4 ==
  data: u input; torque output; a input; b input
function torque = T(u,a,b)    % Guan et al (nonlinear logarithmic equation mentioned in their paper)
    torque = 0;
    if (u >= 0)
     torque= a*(exp(u/2.50)-1)/1.02;

    elseif (u< 0)
     torque= b*(exp(u/-2.58)-1)/(-0.82)   ;
end
